simulink library "AEMS_Standard_Library"  (R2016b)
settings: Solver=ode45  StartTime=0.0  StopTime=10.0  RelTol=1e-3
undefined symbols (not defined in the file or in its folder): BkPY, Cbx_extegr, Cbx_lpegrsys, Cbx_portegr, Cnx_bnk_nr_conf, Cnx_cyl_nr_conf, Cxx_dcm_io_tmr_end_xxxx, Cxx_dcm_rt_tmr_end, Cxx_DID_xxxx_IO_max, Cxx_DID_xxxx_IO_min, Cxx_vmaniegi, DEM_DEBOUNCE_FREEZE, DEM_DTR_CTL_INVISIBLE, DEM_DTR_CTL_NORMAL, Dem_DtrId2_XXX, Dem_DtrId3_XXX, Dem_DtrId4_XXX, Dem_DtrId5_XXX, Dem_DtrId6_XXX, Dem_DtrId7_XXX, Dem_DtrId8_XXX, Dem_DtrId9_XXX, Dem_DtrId_XXX, Dem_EnableConditionId2_XXX, Dem_EnableConditionId3_XXX, Dem_EnableConditionId4_XXX, Dem_EnableConditionId5_XXX, Dem_EnableConditionId6_XXX, Dem_EnableConditionId7_XXX, Dem_EnableConditionId8_XXX, Dem_EnableConditionId_XXX, Dem_EventId, Dem_EventId2_XXX, Dem_EventId3_XXX, Dem_EventId4_XXX, Dem_EventId5_XXX, Dem_EventId6_XXX, Dem_EventId7_XXX, Dem_EventId8_XXX, Dem_EventId9_XXX, Dem_EventId_Device_Faulttype, Dem_EventId_XXX, DEM_IUMPR_GENERAL_DENOMINATOR, DEM_OPCYC_IGNITION, Dem_RatioId2_XXX, Dem_RatioId3_XXX, Dem_RatioId4_XXX, Dem_RatioId5_XXX, Dem_RatioId6_XXX, Dem_RatioId7_XXX, Dem_RatioId8_XXX, Dem_RatioId_XXX, Dem_StorageConditionId2_XXX, Dem_StorageConditionId3_XXX, Dem_StorageConditionId4_XXX, Dem_StorageConditionId5_XXX, Dem_StorageConditionId6_XXX, Dem_StorageConditionId7_XXX, Dem_StorageConditionId8_XXX, Dem_StorageConditionId_XXX ... (+14)
undefined symbols (not defined in the file): BreakPoint, Breakpoint, BreakPoint_X, BreakPoint_Y, Cbx_dem_byp_fail_Device_Faulttype, Cbx_dem_jmp_dwn_act_Device_Faulttype, Cbx_dem_jmp_up_act_Device_Faulttype, Cnx_dem_fail_thd_Device_Faulttype, Cnx_dem_jmp_dwn_ppass_Device_Faulttype, Cnx_dem_jmp_up_pfail_Device_Faulttype, Cnx_dem_pass_thd_Device_Faulttype, Cnx_dem_pfail_inc_step_Device_Faulttype, Cnx_dem_ppass_dec_step_Device_Faulttype, Cxb, Cxb_lb_dly_t_para, Cxb_x, Cxb_X, Cxb_y, Cxb_Y, Cxd, Cxm, Cxp, Cxp_lb_a1_1, Cxp_lb_a1_2, Cxp_lb_a1_3, Cxp_lb_a2_1, Cxp_lb_a2_2, Cxp_lb_a2_3, Cxp_lb_b0_1, Cxp_lb_b0_2, Cxp_lb_b0_3, Cxp_lb_b1_1, Cxp_lb_b1_2, Cxp_lb_b1_3, Cxx_dem_fail_thd_Device_Faulttype, Cxx_dem_pass_thd_Device_Faulttype, Cxx_Tol, Cxx_Tol_X, Cxx_Tol_Y, Nnx_dcm_rt_abrt_stt, Nnx_dcm_rt_run_stt, Nxb_fil_para, Nxp_fil_para
libraries: AEMS_Standard_Library x477, simulink x2
(part 1 of 39)
settings Model: ModifiedComment=z021453 -- Mon Apr 01 17:30:33 2019 -- Version $Revision: 2-12 $\nDebugVer:68  Creator=p075121  LastModifiedBy=a002701
settings Model: ModifiedHistory=|
  | AEMS_Standard_Library_02_15_6: by Etienne, Jegan and Caleb, 08-04-2020
  | 
  | 1.AEMS_Standard_Library/DISCONTINUITIES/AEMS_ENUMERATION_SWITCH: Mask Initialisation code updated to avoid block update for inputs, if DataPortIndices is not available in workspace. Icon Drawing Code Updated
  | 
  | AEMS_Standard_Library_02_15_5: by Caleb and Saravana, 01-04-2020
  | 
  | 1.AEMS_Standard_Library/DISCONTINUITIES/AEMS_ENUMERATION_SWITCH: Mask Initialisation code updated to avoid initial loading warning.
  | 
  | AEMS_Standard_Library_02_15_3: by Sindhuja, 20-03-2020
  | 
  | 1.AEMS_Standard_Library/DISCONTINUITIES/AEMS_ENUMERATION_SWITCH: Mask initialisation code is updated to handle multiple constants for single dataport and mask appearance is modified.
  | 2.AEMS_Standard_Library/SPECIFIC/AEMS_SUPPLIER_CALL_ICLC_LEARNING: New supplier call block for ICLC_LEARNING
  | 
  | AEMS_Standard_Library_02_15_2: by Sindhuja, 09-03-2020
  | 
  | 1.AEMS_Standard_Library/DISCONTINUITIES/AEMS_ENUMERATION_SWITCH: Custom multiport switch block to display enum constant names on the mask.
  | 2.AEMS_Standard_Library/DCM/AEMS_DCM_DID_WRITEDATA:Deletion of NVM WriteOnFly settings.
  | 
  | AEMS_Standard_Library_02_15_1: by Sindhuja, 04-03-2020
  | 
  | 1.Naming convention of Bus Signal wire names are reverted to Uppercase "Index" and "Ratio" [AUTOSAR Constraint] for the below blocks.
  | AEMS_Standard_Library/LOOKUP_TABLES/AEMS_DIRECTLU_1D
  | AEMS_Standard_Library/LOOKUP_TABLES/AEMS_DIRECTLU_2D
  | AEMS_Standard_Library/LOOKUP_TABLES/AEMS_DIRECTLU_INDEXED_1D
  | AEMS_Standard_Library/LOOKUP_TABLES/AEMS_DIRECTLU_INDEXED_2D
  | 
  | 2.To display EventId as eventid in the Attribute format string as per the MXAM guidelines. And added new raster suffix to “DataStoreName” and now the code is generalised to add any type of new raster suffix in the below blocks.
  | AEMS_Standard_Library/DEM/AEMS_DEM_COUNTER_BASED_DEBOUNCE_THRSHOLD_DYN
  | AEMS_Standard_Library/DEM/AEMS_DEM_TIME_BASED_DEBOUNCE_THRSHOLD_DYN
  | 
  | 3.Added new raster suffix to “DataStoreName” and now the code is generalised to add any type of new raster suffix.
  | "AEMS_Standard_Library/SPECIFIC/" : 89 Supplier call blocks
  | AEMS_Standard_Library/SUB/AEMS_DEM_GETEVENTSTATUS
  | AEMS_Standard_Library/SUB/AEMS_FIM_GETFUNCTIONPERMISSION
  | AEMS_Standard_Library/DEM/AEMS_DEM_COUNTER_BASED_DEBOUNCE
  | AEMS_Standard_Library/DEM/AEMS_DEM_TIME_BASED_DEBOUNCE
  | AEMS_Standard_Library_02_15_0: by Sindhuja, 14-02-2020
  | 
  | 1.AEMS_Standard_Library/LOOKUP_TABLES/AEMS_PRE_INTERP: Naming convention of Bus Signal wire names are reverted to Uppercase "Index" and "Ratio" [AUTOSAR Constraint]
  | 
  | To avoid underspecified datatype warnings, stronger typing of the datatypes are done in the below library blocks:
  | 1.AEMS_Standard_Library/DCM/AEMS_APP_REQUEST_ROUTINE:The Output Datatype of the following blocks is strongly typed as "single" in "AEMS_APP_REQUEST_ROUTINE/Timer_routine_Subsystem/" Product,Divide,Sum blocks.
  | 2.AEMS_Standard_Library/DCM/AEMS_DCM_REQUEST_RESULT/Callback_Subsystem/Add:Output Datatype is strongly typed as “uint8”.
  | 3.AEMS_Standard_Library/DCM/AEMS_APP_REQUEST_IOCONTROL/Timer_IOControl_Subsystem/Sum:Output Datatype of the sum block is strongly typed as "single".
  | 4.AEMS_Standard_Library/DCM/AEMS_DCM_START_ROUTINE/Callback_Subsystem/Add:Output Datatype for the above block should be strongly typed as “uint8”.
  | 5.AEMS_Standard_Library/DCM/AEMS_DCM_STOP_ROUTINE/Xxx_Stop_Callback/Add:Output Datatype for the above block is strongly typed as “uint8”.
  | 6.AEMS_Standard_Library/TIMER/AEMS_TIMER1:Output Datatype of the constant blocks are strongly typed as "single" for Constant1,Constant2,Constant3,Constant4,Constant5 blocks.
  | 
  | AEMS_Standard_Library_02_14_2: by Sindhuja, 28-11-2019
  | 
  | 1.AEMS_Standard_Library/LOOKUP_TABLES/AEMS_ITP3D: Block is migrated from RSA_Itp3D for computing 3D interpolation
  | 2.AEMS_Standard_Library/DEM/AEMS_DEM_REP_IUMPR: The background colour of the block is made red as the block is obsolete
  | 3.AEMS_Standard_Library/DCM/AEMS_DCM_DID_WRITEDATA: Optimization of the Mask Initialization code
  | 4.AEMS_Standard_Library/DCM/AEMS_DCM_IO_SHORT_TERM_ADJUSTMENT: Optimization of the Mask Initialization code
  | 5.AEMS_Standard_Library/DEM/AEMS_DEM_SET_EVENT_STS: Default dimension of the block is set as "1“ when the Specific case for Nissan is “on”
  | 6.AEMS_Standard_Library/DEM/AEMS_DEM_SET_DTR: Default dimension of the block is set as "1“ when the Specific case for Nissan is “on”
  | 
  | AEMS_Standard_Library_02_13_13: by Sindhuja, 18-10-2019
  | 
  | 1. AEMS_Standard_Library/DCM/AEMS_DCM_IO_SHORT_TERM_ADJUSTMENT: DataType “Boolean” is added in parameter DID_DataType.
  |   The output datatype of the constant blocks “Cxx_DID_xxxx_IO_max” and “Cxx_DID_xxxx_IO_min” is set to “Inherit via back propagation”.
  | 2. AEMS_Standard_Library/MATH/AEMS_PROTECTED_DIVISION: Block has been updated to take care of vector denominator.
  | 3. Graphical changes(Default size) of these blocks are made as same as that of REMS:
  |    AEMS_Standard_Library/FLAG/AEMS_SRFLIPFLOP
  |    AEMS_Standard_Library/EDGE/AEMS_EDGE_EITHER
  |    AEMS_Standard_Library/EDGE/AEMS_EDGE_FALLING
  |    AEMS_Standard_Library/EDGE/AEMS_EDGE_RISING
  | 
  | AEMS_Standard_Library_02_13_12 : by Smriti, 09-10-2019
  | 
  | 1. AEMS_Standard_Library/DCM/ AEMS_DCM_DID_WRITEDATA: Adding Datatype convert block between “Conversion_Subsystem” blocks and “DID_” blocks.
  | 2. In Data Store Write block, “DataStoreName” is updated according to the “EventId” followed by the raster suffix.
  | AEMS_Standard_Library/DEM/AEMS_DEM_COUNTER_BASED_DEBOUNCE
  | AEMS_Standard_Library/DEM/AEMS_DEM_COUNTER_BASED_DEBOUNCE_THRSHOLD_DYN
  | AEMS_Standard_Library/DEM/AEMS_DEM_TIME_BASED_DEBOUNCE
  | AEMS_Standard_Library/DEM/AEMS_DEM_TIME_BASED_DEBOUNCE_THRSHOLD_DYN
  | 
  | 3. The data type for the constant blocks present in the below listed AEMS blocks is set as "inherit from constant value" for the following blocks:
  | DemDebounceCounterFailedThreshold
  | DemDebounceCounterIncrementStepSize
  | DemDebounceCounterJumpUp
  | DemDebounceCounterJumpUpValue
  | DebounceCounterPassedThreshold
  | DemDebounceCounterDecrementStepSize
  | DemDebounceCounterJumpDown
  | DemDebounceCounterJumpDownValue
  | 
  | AEMS  Library blocks:
  | AEMS_Standard_Library/SUB/AEMS_DEM_COUNTER_BASED_DEBOUNCE_1D
  | AEMS_Standard_Library/SUB/AEMS_DEM_COUNTER_BASED_DEBOUNCE_2D
  | AEMS_Standard_Library/SUB/AEMS_DEM_COUNTER_BASED_DEBOUNCE_3D
  | AEMS_Standard_Library/SUB/AEMS_DEM_COUNTER_BASED_DEBOUNCE_4D
  | AEMS_Standard_Library/SUB/AEMS_DEM_COUNTER_BASED_DEBOUNCE_6D
  | AEMS_Standard_Library/SUB/AEMS_DEM_COUNTER_BASED_DEBOUNCE_8D
  | AEMS_Standard_Library/SUB/AEMS_DEM_COUNTER_BASED_DEBOUNCE_THRSHOLD_DYN_1D
  | AEMS_Standard_Library/SUB/AEMS_DEM_COUNTER_BASED_DEBOUNCE_THRSHOLD_DYN_2D
  | AEMS_Standard_Library/SUB/AEMS_DEM_COUNTER_BASED_DEBOUNCE_THRSHOLD_DYN_3D
  | AEMS_Standard_Library/SUB/AEMS_DEM_COUNTER_BASED_DEBOUNCE_THRSHOLD_DYN_4D
  | AEMS_Standard_Library/SUB/AEMS_DEM_COUNTER_BASED_DEBOUNCE_THRSHOLD_DYN_6D
  | AEMS_Standard_Library/SUB/AEMS_DEM_COUNTER_BASED_DEBOUNCE_THRSHOLD_DYN_8D
  | AEMS_Standard_Library/SUB/AEMS_DEM_TIME_BASED_DEBOUNCE_1D
  | AEMS_Standard_Library/SUB/AEMS_DEM_TIME_BASED_DEBOUNCE_2D
  | AEMS_Standard_Library/SUB/AEMS_DEM_TIME_BASED_DEBOUNCE_3D
  | AEMS_Standard_Library/SUB/AEMS_DEM_TIME_BASED_DEBOUNCE_4D
  | AEMS_Standard_Library/SUB/AEMS_DEM_TIME_BASED_DEBOUNCE_6D
  | 
  | AEMS_Standard_Library_02_13_11 : by Sindhuja, 30-09-2019
  | 
  | 1. AEMS_Standard_Library/MATH/AEMS_COUNTER: The logical implementation has been modified so as to take care when the transition of start_flag from 1 to 0 after saturation occurs at 255.
  | 2. AEMS_Standard_Library/COM/AEMS_FRAME_SUPERVISION:The AEMS_NVM_SET block has been replaced by the unit delay block and vice versa.The Status of the block is sent to unit delay instead of AEMS_NVM_SET in “AEMS_FRAME_SUPERVISION”.
  |     And the Frame_Detected previous value is now sent to AEMS_NVM_SET instead of the unit delay in “AEMS_FRAME_SUPERVISION/ecu_frm_detection”.
  | 3. AEMS_Standard_Library/MEM/AEMS_NVM_WRITEONFLY:Parameter for TriggerType (Rising Edge or Enable) is added.
  |    The  block “AEMS_NVM_WRITEONFLY_ENABLE” is made obsolete.
  | 4. AEMS_Standard_Library/SUB/AEMS_DEM_REPIUMPRDENRELEASE: The attribute format string "sample time" for the "ratioid" is removed.
  |     Dem_RepIUMPRDenLock with the rising edge is removed and the Dem_RepIUMPRDenRelease with the falling edge is replaced with the rising edge in all these blocks.
  |     AEMS_DEM_REP_IUMPR_DEN_RELEASE_1D
  |     AEMS_DEM_REP_IUMPR_DEN_RELEASE_2D
  |     AEMS_DEM_REP_IUMPR_DEN_RELEASE_8D
  | 5. AEMS_Standard_Library/DCM/AEMS_DCM_DID_WRITEDATA: Updated the Initialisation code to set the “TriggerType” of the child library “AEMS_NVM_WRITEONFLY” to “Enable”.
  | 6. AEMS_Standard_Library/DEM/AEMS_FIM_GETFUNCTIONINHIBITION: The constant block “FID_Block” in the below child blocks is set to datatype “uint8”.
  |     AEMS_Standard_Library/SUB/AEMS_FIM_GETFUNCTIONPERMISSION
  |     AEMS_Standard_Library/SUB/AEMS_FIM_GET_FUNC_PMT_1D
  |     AEMS_Standard_Library/SUB/AEMS_FIM_GET_FUNC_PMT_2D
  | 7. AEMS_Standard_Library/SUB/AEMS_FIM_GET_FUNC_PMT_2D: The FIM fid naming has been changed as Fim_fid_xxxx_1 and Fim_fid_xxxx_2
  | 
  | AEMS_Standard_Library_02_13 : by Sindhuja, 18-09-2019
  | 
  | The following blocks are updated with below requirements,
  | -	C**_<Default>_<Faultype> parameters gets updated based on the changes in EventId.
  | -	Additional input “ClearDataRequest” is added.
  | -	New parameter “Cbx_dem_byp_fail_device_faulttype” is added.
  | -	Write output To DataStoreMemory mode added.
  | 
  | 1. AEMS_Standard_Library/DEM/AEMS_DEM_TIME_BASED_DEBOUNCE
  | 2. AEMS_Standard_Library/DEM/AEMS_DEM_COUNTER_BASED_DEBOUNCE
  | 3. AEMS_Standard_Library/DEM/AEMS_DEM_COUNTER_BASED_DEBOUNCE_THRSHOLD_DYN
  | 4. AEMS_Standard_Library/DEM/AEMS_DEM_TIME_BASED_DEBOUNCE_THRSHOLD_DYN
  | 5. AEMS_Standard_Library/SUB/AEMS_DEM_COUNTERBASEDDEBOUNCE
  | 6. AEMS_Standard_Library/SUB/AEMS_DEM_COUNTER_BASED_DEBOUNCE_1D
  | 7. AEMS_Standard_Library/SUB/AEMS_DEM_COUNTER_BASED_DEBOUNCE_2D
  | 8. AEMS_Standard_Library/SUB/AEMS_DEM_COUNTER_BASED_DEBOUNCE_3D
  | 9. AEMS_Standard_Library/SUB/AEMS_DEM_COUNTER_BASED_DEBOUNCE_4D
  | 10. AEMS_Standard_Library/SUB/AEMS_DEM_COUNTER_BASED_DEBOUNCE_6D
  | 11. AEMS_Standard_Library/SUB/AEMS_DEM_COUNTER_BASED_DEBOUNCE_8D
  | 12.AEMS_Standard_Library/SUB/AEMS_DEM_COUNTER_BASED_DEBOUNCE_THRSHOLD_DYN_1D
  | 13.AEMS_Standard_Library/SUB/AEMS_DEM_COUNTER_BASED_DEBOUNCE_THRSHOLD_DYN_2D
  | 14.AEMS_Standard_Library/SUB/AEMS_DEM_COUNTER_BASED_DEBOUNCE_THRSHOLD_DYN_3D
  | 15.AEMS_Standard_Library/SUB/AEMS_DEM_COUNTER_BASED_DEBOUNCE_THRSHOLD_DYN_4D
  | 16.AEMS_Standard_Library/SUB/AEMS_DEM_COUNTER_BASED_DEBOUNCE_THRSHOLD_DYN_6D
  | 17.AEMS_Standard_Library/SUB/AEMS_DEM_COUNTER_BASED_DEBOUNCE_THRSHOLD_DYN_8D
  | 18.AEMS_Standard_Library/SUB/AEMS_DEM_TIMEBASEDDEBOUNCE
  | 19.AEMS_Standard_Library/SUB/AEMS_DEM_TIME_BASED_DEBOUNCE_1D
  | 20.AEMS_Standard_Library/SUB/AEMS_DEM_TIME_BASED_DEBOUNCE_2D
  | 21.AEMS_Standard_Library/SUB/AEMS_DEM_TIME_BASED_DEBOUNCE_3D
  | 22.AEMS_Standard_Library/SUB/AEMS_DEM_TIME_BASED_DEBOUNCE_4D
  | 23.AEMS_Standard_Library/SUB/AEMS_DEM_TIME_BASED_DEBOUNCE_6D
  | 24.AEMS_Standard_Library/SUB/AEMS_DEM_TIME_BASED_DEBOUNCE_8D
  | 25.AEMS_Standard_Library/SUB/AEMS_DEM_TIME_BASED_DEBOUNCE_THRSHOLD_DYN_1D
  | 26.AEMS_Standard_Library/SUB/AEMS_DEM_TIME_BASED_DEBOUNCE_THRSHOLD_DYN_2D
  | 27.AEMS_Standard_Library/SUB/AEMS_DEM_TIME_BASED_DEBOUNCE_THRSHOLD_DYN_3D
  | 28.AEMS_Standard_Library/SUB/AEMS_DEM_TIME_BASED_DEBOUNCE_THRSHOLD_DYN_4D
  | 29.AEMS_Standard_Library/SUB/AEMS_DEM_TIME_BASED_DEBOUNCE_THRSHOLD_DYN_6D
  | 30.AEMS_Standard_Library/SUB/AEMS_DEM_TIME_BASED_DEBOUNCE_THRSHOLD_DYN_8D
  | 
  | 31.AEMS_Standard_Library/DCM/AEMS_DCM_DID_WRITEDATA:
  | -	Parameter name has been changed from “DID Datatype” to “DID Monitoring Datatype”.
  | -	When NVM WriteOnFly Variables is ON, the output of each DID will be tapped into an input of the AEMS_NVM_WRITEONFLY block.
  | -	According to the New rule ARS_STP, the sample time of the constant blocks are set as "inf" in these blocks: AEMS_DCM_DID_WRITEDATA/Callback_Subsystem/..Constant3,
  | 	Constant2, Constant1, NRC1.
  | 
  | 32.AEMS_Standard_Library/MEM/AEMS_NVM_WRITEONFLY: Block is updated to throw an error when the “Number of Inputs” is zero.
  | 33.AEMS_Standard_Library/MATH/AEMS_PROTECTED_DIVISION: New block that replaces the block AEMS_DIVISION_BY_ZERO with a new parameter "Output when |Denominator| < Tolerance".
  |    AEMS_DIVISION_BY_ZERO block is made obsolete. So use AEMS_PROTECTED_DIVISION instead.
  | 34.AEMS_Standard_Library/SUB/AEMS_DEADZONE: The functional implementation has been modified to match REMS behaviour.Block is moved from category "SUB" to "DISCONTINUITIES"
  | 35.AEMS_Standard_Library/DEM/AEMS_DEM_GET_INDICATOR_STS: New parameter for "Simulation Mode" is added.
  | 36.AEMS_Standard_Library/SUB/AEMS_DEM_GETINDICATORSTATUS: New parameter for "Simulation Mode" is added.
  | 37.AEMS_Standard_Library/MATH/AEMS_MATRIX_INVERSION: New block to compute the inversion of a 3*3 matrix.
  | 38.AEMS_Standard_Library/LOOKUP_TABLES/AEMS_INDEXED_LUT_1D_TOL: Newly added block equivalent to RSA_Index_1D_Tol_v01_02
  | 
  | Updated the raster suffix to be added for “DataStoreName” in the “DataStoreRead” block and the constant block “FID block” is set to datatype “uint32” in the below blocks.
  | 39.AEMS_Standard_Library/SUB/AEMS_FIM_GETFUNCTIONPERMISSION
  | 40.AEMS_Standard_Library/SUB/AEMS_FIM_GET_FUNC_PMT_1D
  | 41.AEMS_Standard_Library/SUB/AEMS_FIM_GET_FUNC_PMT_2D
  | 42.AEMS_Standard_Library/DEM/AEMS_FIM_GETFUNCTIONINHIBITION
  | 
  | 43."AEMS_Standard_Library/SPECIFIC/" : 89 Supplier call blocks are updated  under this category: The raster suffix gets added for the “DataStoreName” in the “DataStoreRead” block with respect to the function call trigger.
  | 44.AEMS_Standard_Library/SAFETY/AEMS_SAFETY_AND_REGULATION: To insure traceability of Safety and Regulation requirements, new block AEMS_SAFETY_AND_REGULATION is added.
  | 
  | The parameter case has been changed from Dem_StorageConditionID to "Dem_StorageConditionId" in the below blocks.
  | 45.AEMS_Standard_Library/DEM/AEMS_DEM_SET_STORAGE_COND
  | 46.AEMS_Standard_Library/SUB/AEMS_DEM_SET_STORAGE_COND_2D
  | 47.AEMS_Standard_Library/DEM/AEMS_DEM_SET_STORAGE_COND_3D
  | 48.AEMS_Standard_Library/DEM/AEMS_DEM_SET_STORAGE_COND_8D
  | 
  | 49.AEMS_Standard_Library/DCM/AEMS_DCM_IO_SHORT_TERM_ADJUSTMENT: Block spelling is corrected from AEMS_DCM_IO_SHORT_TERM_ADJUSTEMENT to AEMS_DCM_IO_SHORT_TERM_ADJUSTMENT
  | 50.AEMS_Standard_Library/SUB/AEMS_SORT_MEDIAN: "AEMS_SORT_MEDIAN/Pair/Add1" here "Require all inputs to have same datatype" and "Saturate on integer overflow" has been enabled.
  | 51.AEMS_Standard_Library/DISCRETE/AEMS_UNITDELAY_RESET_EXTERNALIC: The wire names has been removed for inports 2 and 3.
  | 52.AEMS_Standard_Library/FILTER/AEMS_FIRST_ORDER_FILTER_RST: Stronger typing of DataTypes of Sum, Sum1, Product1 and Product2 blocks are changed to “single” to avoid warnings.
  | 
  | 
  | AEMS_Standard_Library_02_12 : by Sindhuja, 21-06-2019
  | 
  | New parameter "Function Mode" is added for DSM possibility in the following blocks:
  | 1. AEMS_Standard_Library/DEM/AEMS_DEM_GET_EVENT_STS
  | 2. AEMS_Standard_Library/SUB/AEMS_DEM_GETEVENTSTATUS
  | 3. AEMS_Standard_Library/SUB/AEMS_DEM_GET_EVENT_STS_1D
  | 4. AEMS_Standard_Library/SUB/AEMS_DEM_GET_EVENT_STS_2D
  | 5. AEMS_Standard_Library/SUB/AEMS_DEM_GET_EVENT_STS_8D
  | 6. AEMS_Standard_Library/SUB/AEMS_DEM_GET_EVENT_STS_9D
  | 
  | 7. AEMS_Standard_Library/BIT_OPERATION/AEMS_BIT_SET32: New Library block
  | 
  | 8. AEMS_Standard_Library/MATH/AEMS_SORT: New Library block to sort one-dimensional arrays
  | 9. AEMS_Standard_Library/SUB /AEMS_SORT_MEDIAN: Child library for AEMS_SORT, to get the median vector after sorting the N numbers in ascending order.
  | 
  | 10. AEMS_Standard_Library/MATH/AEMS_SORT:Implementation has been modified in "AEMS_SORT/For_loop_1/For_loop_2/Unit_delay_vector"
  | 
  | AEMS_Standard_Library_02_12 : by Sindhuja, 06-06-2019
  | "Dem debounce behavior 1" is set to "DEM_DEBOUNCE_FREEZE" by default for the following blocks:
  | 1. AEMS_Standard_Library/DEM/AEMS_DEM_TIME_BASED_DEBOUNCE
  | 2. AEMS_Standard_Library/DEM/AEMS_DEM_COUNTER_BASED_DEBOUNCE
  | 3. AEMS_Standard_Library/DEM/AEMS_DEM_TIME_BASED_DEBOUNCE_THRSHOLD_DYN
  | 
  | 4. AEMS_Standard_Library/SUB/AEMS_DEM_SET_STORAGE_COND_1D: The Output Datatype of StorageCondId is set to uint8
  | 5. AEMS_Standard_Library/SUB/AEMS_DEM_REP_IUMPR_1D: The Output Datatype of RatioId is set to uint16
  | 6. AEMS_Standard_Library/SUB/AEMS_DEM_REP_IUMPR_2D: The Output Datatype of RatioId is set to uint16
  | 7. AEMS_Standard_Library/SUB/AEMS_DEM_REP_IUMPR_DEN_RELEASE_1D: The Output Datatype of RatioId is set to uint16
  | 8. AEMS_Standard_Library/SUB/AEMS_DEM_REP_IUMPR_DEN_RELEASE_2D: The Output Datatype of RatioId is set to uint16
  | 9. AEMS_Standard_Library/SUB/AEMS_DEM_REP_IUMPR_FAULTDETECT_1D: The Output Datatype of RatioId is set to uint16
  | 10. AEMS_Standard_Library/SUB/AEMS_DEM_REP_IUMPR_FAULTDETECT_2D: The Output Datatype of RatioId is set to uint16
  | 11. AEMS_Standard_Library/SUB/AEMS_DEM_SET_EVENT_DSBL_1D: The Output Datatype of EventId is set to uint16
  | 12. AEMS_Standard_Library/SUB/AEMS_DEM_GET_EVENT_STS_1D: The Output Datatype of EventId is set to uint16
  | 
  | 
  | AEMS_Standard_Library_02_12 : by Sindhuja, 24-05-2019
  | 1.AEMS_Standard_Library/MATH/AEMS_SQRT: Added option for reciprocal square root in the "Function of Sqrt"
  | 2.AEMS_Standard_Library/DEM/AEMS_FIM_GETFUNCTIONINHIBITION: Updated AEMS_FIM_GetFunctionInhibition to add DSM possibility
  | 3.AEMS_Standard_Library/SUB/AEMS_FIM_GETFUNCTIONPERMISSION: Added DSM possibility
  | 4.AEMS_Standard_Library/SUB/AEMS_FIM_GET_FUNC_PMT_1D: Added DSM possibility
  | 5.AEMS_Standard_Library/SUB/AEMS_FIM_GET_FUNC_PMT_2D: Added DSM possibility
  | 6.New blocks migrated from NEMS to "AEMS_Standard_Library/SPECIFIC"
  |  AEMS_AIR_BALANCE
  |  AEMS_BACK_UP
  |  AEMS_BACK_UP_AVE
  |  AEMS_BACKUP_FOR_ENGINE_OFF_MONITOR
  |  AEMS_DGNDMDPGCUT
  |  AEMS_DGN_MF_MISX_CALCULATION_LIB
  |  AEMS_UL_INTERP
  |  AEMS_INTERP_WITH_BREAKPOINT
  |  AEMS_LOOKUP_LIBRARY
  |  AEMS_EGR_OFFSET_BLOCK_DIM8
  |  AEMS_EGR_RATE_TRANSPORTOR_LIB
  |  AEMS_OL_RATE_COUNTER
  |  AEMS_OL_SIMILAR_CONDITION_SET
  |  AEMS_STATE_TRANSITION_SET_VALUE
  |  AEMS_OL_RATE_COUNTER_B
  |  AEMS_OL_SIMILAR_CONDITION_CHECK
  |  AEMS_EGR_RESPONSE_TIME_CAL_LIB
  |  AEMS_EGRQESTH_SELECT_AND_TRIM_LIB
  |  AEMS_DGN_BB_RESULT
  | 
  |  7.EventId Numbering changed for the below blocks:
  |  AEMS_Standard_Library/SUB/AEMS_DEM_COUNTER_BASED_DEBOUNCE_THRSHOLD_DYN_2D
  |  AEMS_Standard_Library/SUB/AEMS_DEM_COUNTER_BASED_DEBOUNCE_THRSHOLD_DYN_3D
  |  AEMS_Standard_Library/SUB/AEMS_DEM_COUNTER_BASED_DEBOUNCE_THRSHOLD_DYN_4D
  |  AEMS_Standard_Library/SUB/AEMS_DEM_COUNTER_BASED_DEBOUNCE_THRSHOLD_DYN_6D
  |  AEMS_Standard_Library/SUB/AEMS_DEM_COUNTER_BASED_DEBOUNCE_THRSHOLD_DYN_8D
  |  AEMS_Standard_Library/SUB/AEMS_DEM_TIME_BASED_DEBOUNCE_THRSHOLD_DYN_2D
  |  AEMS_Standard_Library/SUB/AEMS_DEM_TIME_BASED_DEBOUNCE_THRSHOLD_DYN_3D
  |  AEMS_Standard_Library/SUB/AEMS_DEM_TIME_BASED_DEBOUNCE_THRSHOLD_DYN_4D
  |  AEMS_Standard_Library/SUB/AEMS_DEM_TIME_BASED_DEBOUNCE_THRSHOLD_DYN_6D
  |  AEMS_Standard_Library/SUB/AEMS_DEM_TIME_BASED_DEBOUNCE_THRSHOLD_DYN_8D
  |  AEMS_Standard_Library/SUB/AEMS_DEM_TIME_BASED_DEBOUNCE_2D
  |  AEMS_Standard_Library/SUB/AEMS_DEM_TIME_BASED_DEBOUNCE_3D
  |  AEMS_Standard_Library/SUB/AEMS_DEM_TIME_BASED_DEBOUNCE_4D
  |  AEMS_Standard_Library/SUB/AEMS_DEM_TIME_BASED_DEBOUNCE_6D
  |  AEMS_Standard_Library/SUB/AEMS_DEM_TIME_BASED_DEBOUNCE_8D
  |  AEMS_Standard_Library/SUB/AEMS_DEM_COUNTER_BASED_DEBOUNCE_2D
  |  AEMS_Standard_Library/SUB/AEMS_DEM_COUNTER_BASED_DEBOUNCE_3D
  |  AEMS_Standard_Library/SUB/AEMS_DEM_COUNTER_BASED_DEBOUNCE_4D
  |  AEMS_Standard_Library/SUB/AEMS_DEM_COUNTER_BASED_DEBOUNCE_6D
  |  AEMS_Standard_Library/SUB/AEMS_DEM_COUNTER_BASED_DEBOUNCE_8D
  |  AEMS_Standard_Library/SUB/AEMS_DEM_SET_STORAGE_COND_2D
  |  AEMS_Standard_Library/SUB/AEMS_DEM_SET_STORAGE_COND_8D
  |  AEMS_Standard_Library/SUB/AEMS_DEM_REP_IUMPR_2D
  |  AEMS_Standard_Library/SUB/AEMS_DEM_REP_IUMPR_8D
  |  AEMS_Standard_Library/SUB/AEMS_DEM_REP_IUMPR_DEN_RELEASE_2D
  |  AEMS_Standard_Library/SUB/AEMS_DEM_REP_IUMPR_DEN_RELEASE_8D
  |  AEMS_Standard_Library/SUB/AEMS_DEM_REP_IUMPR_FAULTDETECT_2D
  |  AEMS_Standard_Library/SUB/AEMS_DEM_REP_IUMPR_FAULTDETECT_8D
  |  AEMS_Standard_Library/SUB/AEMS_DEM_SET_EVENT_DSBL_2D
  |  AEMS_Standard_Library/SUB/AEMS_DEM_SET_EVENT_DSBL_8D
  |  AEMS_Standard_Library/SUB/AEMS_DEM_SET_EVENT_DSBL_9D
  |  AEMS_Standard_Library/SUB/AEMS_DEM_GET_EVENT_STS_2D
  |  AEMS_Standard_Library/SUB/AEMS_DEM_GET_EVENT_STS_8D
  |  AEMS_Standard_Library/SUB/AEMS_DEM_GET_EVENT_STS_9D
  |  AEMS_Standard_Library/SUB/AEMS_DEM_SET_EVENT_STS_2D
  |  AEMS_Standard_Library/SUB/AEMS_DEM_SET_EVENT_STS_8D
  |  AEMS_Standard_Library/SUB/AEMS_DEM_SET_EVENT_STS_9D
  |  AEMS_Standard_Library/SUB/AEMS_DEM_SET_EVENT_AVL_2D
  |  AEMS_Standard_Library/SUB/AEMS_DEM_SET_EVENT_AVL_8D
  |  AEMS_Standard_Library/SUB/AEMS_DEM_SET_EVENT_AVL_9D
  |  AEMS_Standard_Library/SUB/AEMS_FIM_GET_FUNC_PMT_2D
  |  AEMS_Standard_Library/SUB/AEMS_DEM_SET_ENBL_COND_2D
  |  AEMS_Standard_Library/SUB/AEMS_DEM_SET_ENBL_COND_8D
  |  AEMS_Standard_Library/SUB/AEMS_DEM_SET_DTR_2DS
  |  AEMS_Standard_Library/SUB/AEMS_DEM_SET_DTR_8DS
  |  AEMS_Standard_Library/SUB/AEMS_DEM_SET_DTR_2DU
  |  AEMS_Standard_Library/SUB/AEMS_DEM_SET_DTR_8DU
  |  AEMS_Standard_Library/SUB/AEMS_DEM_SET_DTR_9DU
  | 
  |  8.Changed EventID to EventId in the below blocks:
  |  AEMS_Standard_Library/DEM/AEMS_DEM_SET_EVENT_AVL
  |  AEMS_Standard_Library/DEM/AEMS_DEM_TIME_BASED_DEBOUNCE
  |  AEMS_Standard_Library/DEM/AEMS_DEM_COUNTER_BASED_DEBOUNCE
  |  AEMS_Standard_Library/DEM/AEMS_DEM_TIME_BASED_DEBOUNCE_THRSHOLD_DYN
  |  AEMS_Standard_Library/DEM/AEMS_DEM_COUNTER_BASED_DEBOUNCE_THRSHOLD_DYN
  |  AEMS_Standard_Library/SUB/AEMS_DEM_TIMEBASEDDEBOUNCE
  |  AEMS_Standard_Library/SUB/AEMS_DEM_COUNTERBASEDDEBOUNCE
  |  AEMS_Standard_Library/SUB/AEMS_DEM_COUNTER_BASED_DEBOUNCE_THRSHOLD_DYN_1D
  |  AEMS_Standard_Library/SUB/AEMS_DEM_COUNTER_BASED_DEBOUNCE_THRSHOLD_DYN_2D
  |  AEMS_Standard_Library/SUB/AEMS_DEM_COUNTER_BASED_DEBOUNCE_THRSHOLD_DYN_3D
  |  AEMS_Standard_Library/SUB/AEMS_DEM_COUNTER_BASED_DEBOUNCE_THRSHOLD_DYN_4D
  |  AEMS_Standard_Library/SUB/AEMS_DEM_COUNTER_BASED_DEBOUNCE_THRSHOLD_DYN_6D
  |  AEMS_Standard_Library/SUB/AEMS_DEM_COUNTER_BASED_DEBOUNCE_THRSHOLD_DYN_8D
  |  AEMS_Standard_Library/SUB/AEMS_DEM_TIME_BASED_DEBOUNCE_THRSHOLD_DYN_1D
  |  AEMS_Standard_Library/SUB/AEMS_DEM_TIME_BASED_DEBOUNCE_THRSHOLD_DYN_2D
  |  AEMS_Standard_Library/SUB/AEMS_DEM_TIME_BASED_DEBOUNCE_THRSHOLD_DYN_3D
  |  AEMS_Standard_Library/SUB/AEMS_DEM_TIME_BASED_DEBOUNCE_THRSHOLD_DYN_4D
  |  AEMS_Standard_Library/SUB/AEMS_DEM_TIME_BASED_DEBOUNCE_THRSHOLD_DYN_6D
  |  AEMS_Standard_Library/SUB/AEMS_DEM_TIME_BASED_DEBOUNCE_THRSHOLD_DYN_8D
  |  AEMS_Standard_Library/SUB/AEMS_DEM_TIME_BASED_DEBOUNCE_1D
  |  AEMS_Standard_Library/SUB/AEMS_DEM_TIME_BASED_DEBOUNCE_2D
  |  AEMS_Standard_Library/SUB/AEMS_DEM_TIME_BASED_DEBOUNCE_3D
  |  AEMS_Standard_Library/SUB/AEMS_DEM_TIME_BASED_DEBOUNCE_4D
  |  AEMS_Standard_Library/SUB/AEMS_DEM_TIME_BASED_DEBOUNCE_6D
  |  AEMS_Standard_Library/SUB/AEMS_DEM_TIME_BASED_DEBOUNCE_8D
  |  AEMS_Standard_Library/SUB/AEMS_DEM_COUNTER_BASED_DEBOUNCE_1D
  |  AEMS_Standard_Library/SUB/AEMS_DEM_COUNTER_BASED_DEBOUNCE_2D
  |  AEMS_Standard_Library/SUB/AEMS_DEM_COUNTER_BASED_DEBOUNCE_3D
  |  AEMS_Standard_Library/SUB/AEMS_DEM_COUNTER_BASED_DEBOUNCE_4D
  |  AEMS_Standard_Library/SUB/AEMS_DEM_COUNTER_BASED_DEBOUNCE_6D
  |  AEMS_Standard_Library/SUB/AEMS_DEM_COUNTER_BASED_DEBOUNCE_8D
  | 
  | 9.AEMS_Standard_Library/LOOKUP_TABLES/AEMS_PRE_INTERP:Naming of the wires is made to lower case
  | 10.AEMS_Standard_Library/SUB/AEMS_DEM_READDATAOFPID01:Signal name “vPID01” is removed inside the library block
  | 11.AEMS_Standard_Library/SUB/AEMS_DEM_SET_DTR_1DU: The Output Datatype for the constant blocks DEM_DTR_CTL_NORMAL & DEM_DTR_CTL_INVISIBLE is changed from "inherit from constant value" to “uint8”
  | 12.AEMS_Standard_Library/SUB/AEMS_DEM_SET_DTR_2DU: The Output Datatype for the constant blocks DEM_DTR_CTL_NORMAL & DEM_DTR_CTL_INVISIBLE is changed from "inherit from constant value" to “uint8”
  | 13.AEMS_Standard_Library/TIMER/AEMS_TIMER: No functional changes. Stronger typing of Datatypes to avoid Underspecified warnings.
  | 14.AEMS_Standard_Library/DCM/AEMS_DCM_IO_SHORT_TERM_ADJUSTEMENT:  The parameter DataSize is replaced by DataType(int8/uint8/int16/uint16/int32/uint32).
  |      Changes done in the “Mask initialization” for the replace block command. A demux block is added to handle if buffer size is 2byte or 4byte.
  | 15.AEMS_Standard_Library/DCM/AEMS_DCM_DID_WRITEDATA:Input is removed and Ground is added.
  | 16.AEMS_Standard_Library/SAFETY/AEMS_FSL_RAM_QM_TO_ASIL: Nissan Safety block
  | 17.AEMS_Standard_Library/SAFETY/AEMS_FSL_RAM_ASIL_TO_QM: Nissan Safety block
  | 18.AEMS_Standard_Library/FILTER/AEMS_TAU_TO_FILTER_PARAM_EXP: An obsolete block for Prefilter with exponential.
  | 
  | AEMS_Standard_Library_02_11 : by Sindhuja, 18-03-2019
  | 1. AEMS_Standard_Library/SUB/AEMS_CONVERT_BUFFER_TO_FLP: Data Type Conversion block added in the library block "AEMS_CONVERT_BUFFER_TO_FLP".
  | 2. AEMS_Standard_Library/DCM/AEMS_DCM_DID_WRITEDATA: Updated the child library block "AEMS_CONVERT_BUFFER_TO_FLP" in "AEMS_DCM_DID_WRITEDATA".
  | 3. AEMS_Standard_Library/DCM/AEMS_FLOAT_TO_FXP: Internal implementation doesn’t have Min/Max Limits. And the parameter "ByteSize" has been changed to "Output Fixed Point datatype".
  | 4. AEMS_Standard_Library/DCM/AEMS_FLOAT_TO_FXP_WITH_LIMIT: Internal implementation has Min/Max Limits. And the parameter "ByteSize" has been changed to "Output Fixed Point datatype".
  | 5. AEMS_Standard_Library/DCM/AEMS_FXP_TO_FLOAT: Data Type Conversion block is added in the implementation to take care of floating resolution.
  | 6. AEMS_Standard_Library/BIT_OPERATION/AEMS_CONVERT_TO_UNSIGNED_SI: New Block is added to convert signed integers to unsigned integers.
  | 7. AEMS_Standard_Library/BIT_OPERATION/AEMS_EXTRACT_BIT: New child library AEMS_CONVERT_TO_UNSIGNED_SI will be added if the Input data type is a signed integer.
  | 8. AEMS_Standard_Library/DCM/AEMS_TO_FXP_WITH_LIMIT: The parameter ‘Byte Size’ is replaced with ‘Output Fixed Point Datatype’ and a Data Type Conversion block is added at the input side.
  | 9. AEMS_Standard_Library/DEM/AEMS_DEM_REP_IUMPR_DEN_RELEASE & AEMS_Standard_Library/DEM/AEMS_DEM_REP_IUMPR_FAULTDETECT: AEMS_DEM_IUMPR block is split as two blocks.
  |    The following child library blocks in "AEMS_Standard_Library/SUB"
  |    AEMS_DEM_REP_IUMPR_DEN_RELEASE_1D
  |    AEMS_DEM_REP_IUMPR_DEN_RELEASE_2D
  |    AEMS_DEM_REP_IUMPR_DEN_RELEASE_8D
  |    AEMS_DEM_REP_IUMPR_FAULTDETECT_1D
  |    AEMS_DEM_REP_IUMPR_FAULTDETECT_2D
  |    AEMS_DEM_REP_IUMPR_FAULTDETECT_8D
  | 10. AEMS_Standard_Library/DCM/AEMS_DCM_DID_READDATA: Updated the block to read signed FXP. Parameter changed from Byte Size to DataType.
  | 11. AEMS_Standard_Library/DCM/AEMS_DCM_DID_WRITEDATA: Updated the block to support negative values & Existing bugs were removed. Parameter changed from Byte Size to DataType.
  | 12. AEMS_Standard_Library/SUB/AEMS_CONVERT_BUFFER_TO_FLP: Updated the block to support negative integer values. Parameter “Byte Size” changed to “DIDType”.
  | 13. AEMS_Standard_Library/SUB/AEMS_CONVERT_BYTE_TO_FLP: A new block created to convert byte data to float data, based on the resolution and offset.
  | 14. New blocks: (By Etienne)
  |        AEMS_Standard_Library/SUB/AEMS_DEM_SET_DTR_9DU
  |        AEMS_Standard_Library/SUB/AEMS_DEM_SET_EVENT_DSBL_9D
  |        AEMS_Standard_Library/SUB/AEMS_DEM_GET_EVENT_STS_9D
  |        AEMS_Standard_Library/SUB/AEMS_DEM_SET_EVENT_STS_9D
  |        AEMS_Standard_Library/SUB/AEMS_DEM_SET_EVENT_AVL_9D
  | 
  | 15. Modified blocks: (By Etienne)
  |        AEMS_Standard_Library/DEM/AEMS_DEM_READ_DATA_PID01
  |        AEMS_Standard_Library/DEM/AEMS_DEM_SET_DTR
  |        AEMS_Standard_Library/DEM/AEMS_DEM_SET_EVENT_DSBL
  |        AEMS_Standard_Library/DEM/AEMS_DEM_GET_EVENT_STS
  |        AEMS_Standard_Library/DEM/AEMS_DEM_SET_EVENT_STS
  |        AEMS_Standard_Library/DEM/AEMS_DEM_SET_EVENT_AVL
  |        AEMS_Standard_Library/SUB/AEMS_DEM_SET_EVENT_AVL_1D
  |        AEMS_Standard_Library/SUB/AEMS_DEM_SET_EVENT_AVL_2D
  |        AEMS_Standard_Library/SUB/AEMS_DEM_SET_EVENT_AVL_8D
  | 
  | 
  | 
  | AEMS_Standard_Library_02_10: by Thilagavathi, 11-12-2018
  | 1. Reversed the order of byte for the block "AEMS_DCM_DID_WRITEDATA" in the path "AEMS_Standard_Library/DCM/AEMS_DCM_DID_WRITEDATA"
  | 2. A new block added in the path "AEMS_Standard_Library/SPECIFIC/AEMS_SlopeSwitchExtern"
  | 3. Updated the constnat block parameter for the block "AEMS_INTERP" in the path "AEMS_Standard_Library/LOOKUP_TABLES/AEMS_INTERP"
  | 4. Added the Mask parameter(function mode) for the blocks "AEMS_FIM_GETFUNCTIONINHIBITION, AEMS_FIM_GET_FUNC_PMT_1D, AEMS_FIM_GET_FUNC_PMT_2D & AEMS_FIM_GETFUNCTIONPERMISSION"
  |     in the following path "AEMS_Standard_Library/DEM/AEMS_FIM_GETFUNCTIONINHIBITION" & "AEMS_Standard_Library/SUB/"
  | 5. Upadted data type for 18 Supplier call blocks in the path "AEMS_Standard_Library/SPECIFIC"
  | 6. Attribute string formate changed for the block "AEMS_DEM_COUNTER_BASED_DEBOUNCE" in path "AEMS_Standard_Library/DEM/AEMS_DEM_COUNTER_BASED_DEBOUNCE"
  | 7. Attribute string formate changed for the block "AEMS_DEM_TIME_BASED_DEBOUNCE" in path "AEMS_Standard_Library/DEM/AEMS_DEM_TIME_BASED_DEBOUNCE"
  | 8. changed the subsystem "DEM_SET_EVENT_AVL_E as atomic unit" for block "AEMS_DEM_SET_EVENT_AVL_1D" in the path "AEMS_Standard_Library/SUB/AEMS_DEM_SET_EVENT_AVL_1D"
  | 9. changed the subsystem "DEM_SET_EVENT_AVL_E as atomic unit" for block "AEMS_DEM_SET_EVENT_AVL_2D" in the path "AEMS_Standard_Library/SUB/AEMS_DEM_SET_EVENT_AVL_2D"
  | 10. changed the subsystem "DEM_SET_EVENT_AVL_E as atomic unit" for block "AEMS_DEM_SET_EVENT_AVL_8D" in the path "AEMS_Standard_Library/SUB/AEMS_DEM_SET_EVENT_AVL_8D"
  | 11. A new block "AEMS_FRAME_SUPERVISION" added in the path "AEMS_Standard_Library/COM/AEMS_FRAME_SUPERVISION"
  | 12. updated the block “AEMS_TIMER_H” to avoid the issue(“when timer is start incrementing / decrementing it is not taking the updated target counter value”) in AEMS_DEM_TIME_BASED_DEBOUNCE_THRSHOLD_DYN
  |      in the path "AEMS_Standard_Library/TIMER/AEMS_TIMER_H"
  | 13. Updated blocks "AEMS_DEM_TIME_BASED_DEBOUNCE_THRSHOLD_DYN & AEMS_DEM_COUNTER_BASED_DEBOUNCE_THRSHOLD_DYN" are added in the path "AEMS_Standard_Library/DEM"
  | 14. The following new blocks are added in the path "AEMS_Standard_Library/SUB"
  |       AEMS_DEM_TIME_BASED_DEBOUNCE_THRSHOLD_DYN_1D
  |       AEMS_DEM_TIME_BASED_DEBOUNCE_THRSHOLD_DYN_2D
  |       AEMS_DEM_TIME_BASED_DEBOUNCE_THRSHOLD_DYN_3D
  |       AEMS_DEM_TIME_BASED_DEBOUNCE_THRSHOLD_DYN_4D
  |       AEMS_DEM_TIME_BASED_DEBOUNCE_THRSHOLD_DYN_6D
  |       AEMS_DEM_TIME_BASED_DEBOUNCE_THRSHOLD_DYN_8D
  |       AEMS_DEM_COUNTER_BASED_DEBOUNCE_THRSHOLD_DYN_1D
  |       AEMS_DEM_COUNTER_BASED_DEBOUNCE_THRSHOLD_DYN_2D
  |       AEMS_DEM_COUNTER_BASED_DEBOUNCE_THRSHOLD_DYN_3D
  |       AEMS_DEM_COUNTER_BASED_DEBOUNCE_THRSHOLD_DYN_4D
  |       AEMS_DEM_COUNTER_BASED_DEBOUNCE_THRSHOLD_DYN_6D
  |       AEMS_DEM_COUNTER_BASED_DEBOUNCE_THRSHOLD_DYN_8D
  | 15. Updated the block "AEMS_DCM_DID_WRITEDATA" (replaced the block AEMS_NVM_WRITEONFLY by AEMS_NVM_WRITEONFLY_ENABLE) in the path "AEMS_Standard_Library/DCM/AEMS_DCM_DID_WRITEDATA"
  | 16. A new block "AEMS_NVM_WRITEONFLY_ENABLE" added in the path "AEMS_Standard_Library/MEM/AEMS_NVM_WRITEONFLY_ENABLE"
  | 17. A new block added in the path "AEMS_Standard_Library/COM/AEMS_REQUEST_COUNTER_SWITCH" (migrated from REMS)
  | 18. A new block added in the path "AEMS_Standard_Library/COM/AEMS_REQUEST_COUNTER" (migrated from REMS)
  | 
  | 
  | AEMS_Standard_Library_02_09: by Thilagavathi, 30-08-2018
  | 1. 84 Supplier call blocks are Migrated from REMS (SUPP_CALL_TQ_LIM, SUPPLIER_CALL_FFW & SUPPLIER_CALL_TIM category) and added in the path "AEMS_Standard_Library/SPECIFIC/"
  | 2. Reversed the order of byte for the block "AEMS_DCM_DID_READDATA" in the path "AEMS_Standard_Library/DCM/AEMS_DCM_DID_READDATA"
  | 3. The sample time is changed as '-1' for the block "AEMS_DEM_SET_EVENT_AVL" in the path "AEMS_Standard_Library/DEM/AEMS_DEM_SET_EVENT_AVL"
  | 4. A new block added in the path "AEMS_Standard_Library/DCM/AEMS_DCM_GETSESCTRLTYPE"
  | 5. A new block added in the path "AEMS_Standard_Library/MATH/AEMS_SQRT"
  | 
  | AEMS_Standard_Library_02_08: by Prabhakaran, 30-07-2018
  | 1. Update parameter Duration of Timer in miliseconde for block  in the path "AEMS_Standard_Library/DCM/AEMS_APP_REQUEST_IOCONTROL"
  | 2. Update parameter Duration of Timer (in seconde) for block  in the path "AEMS_Standard_Library/DCM/AEMS_APP_REQUEST_ROUTINE"
  | 3. The following supplier call block are added in the path "AEMS_Standard_Library/SPECIFIC/".
  |  - AEMS_SUPPLIER_CALL_ESTI_TIME_INJ
  |  - AEMS_SUPPLIER_CALL_FUEL_INJ_MIN
  |  - AEMS_SUPPLIER_CALL_PHI_MIN_ING
  |  - AEMS_SUPPLIER_CALL_SEPERATION_MIN_TIME
  |  - AEMS_SUPPLIER_CALL_TI_MIN_OK
  | 4. The following library blocks moved from DISCONTINUITIES to SPECIFIC Category as requiested by Naveen & NML
  |  - AEMS_AT_EHR - "AEMS_Standard_Library/DISCONTINUITIES/AEMS_AT_EHR"
  |  - AEMS_MULTIPORT_TIMESWITCH_CONFIG - "AEMS_Standard_Library/DISCONTINUITIES/AEMS_MULTIPORT_TIMESWITCH_CONFIG"
  |  - AEMS_AT_TUBE - "AEMS_Standard_Library/DISCONTINUITIES/AEMS_AT_TUBE"
  | 
  | AEMS_Standard_Library_02_07: by Thilagavathi, 17-07-2018
  | - A new block added in the path "AEMS_Standard_Library/DISCONTINUITIES/AEMS_AS_PADE"
  | - The block parameter 'DisableCoverage' is set to OFF in the following blocks to enable the coloring option while taking coverage.
  |   1. AEMS_Standard_Library/DISCRETE/AEMS_UNITDELAY_RESET_EXTERNALIC/FixPt_Logical_Operator,
  |   2. AEMS_Standard_Library/DISCRETE/AEMS_UNITDELAY_RESET_EXTERNALIC/FixPt_Logical_Operator1.
  | -A new block added in the path "AEMS_Standard_Library/DISCONTINUITIES/AEMS_AT_EHR"
  | -A new block added in the path "AEMS_Standard_Library/DISCONTINUITIES/AEMS_MULTIPORT_TIMESWITCH_CONFIG"
  | -A new block added in the path "AEMS_Standard_Library/DISCONTINUITIES/AEMS_AT_TUBE"
  | 
  | AEMS_Standard_Library_02_06: by Van-Cuong NGUYEN, 17-05-2018
  | 
  | AEMS_Standard_Library_02_05: by Van-Cuong NGUYEN, 27-03-2018
  | AEMS_Standard_Library/FILTER/AEMS_TAU_TO_FILTER_PARAM: Add block convert time constant to filter parameter, this is only used for filter block
  | AEMS_Standard_Library/DCM/AEMS_API_SUPPLIER_CALL: Add block API Supplier Call to use as interface with Supplier layer. It is not a functionnal block.
  | AEMS_Standard_Library/DCM/AEMS_TO_FXP_WITH_LIMIT: Change option convert from <<round>> to <<floor>> to respect MBDR.
  | AEMS_Standard_Library/DEM/AEMS_DEM_COUNTER_BASED_DEBOUNCE: Update parameter EventId such that block simulate without defining this parameter in workspace.
  | AEMS_Standard_Library/DEM/AEMS_DEM_COUNTER_BASED_DEBOUNCE_THRSHOLD_DYN: Update parameter EventId such that block simulate without defining this parameter in workspace.
  | AEMS_Standard_Library/DEM/AEMS_DEM_TIME_BASED_DEBOUNCE: Update parameter EventId such that block simulate without defining this parameter in workspace.
  | AEMS_Standard_Library/DEM/AEMS_DEM_TIME_BASED_DEBOUNCE_THRSHOLD_DYN: Update parameter EventId such that block simulate without defining this parameter in workspace.
  | AEMS_Standard_Library/DEM/AEMS_DEM_SET_EVENT_AVL: Update parameter EventId such that block simulate without defining this parameter in workspace.
  | 
  | AEMS_Standard_Library_02_04: by Van-Cuong NGUYEN, 14-03-2018
  | AEMS_DEM_TIME_BASED_DEBOUNCE_THRSHOLD_DYN: add in DEM category new block for time based debounce with threshold dynamic and for Nissan uses only
  | AEMS_DEM_COUNTER_BASED_DEBOUNCE_THRSHOLD_DYN: add in DEM category new block for counter based debounce with threshold dynamic and for Nissan uses only
  | AEMS_DCM_DID_READDATA: correct problem of simulation for inport boolean and add inport name in mask for each inport
  | AEMS_DCM_DID_WRITEDATA: correct problem of simulation for inport boolean and add inport name in mask for each inport
  | 
  | AEMS_Standard_Library_02_03: by Van-Cuong NGUYEN, 06-02-2018
  | DEM Blocks
  | AEMS_Standard_Library/DEM/AEMS_DEM_GET_INDICATOR_STS
  | AEMS_Standard_Library/DEM/AEMS_DEM_READ_DATA_PID01
  | AEMS_Standard_Library/DEM/AEMS_DEM_REP_IUMPR
  | AEMS_Standard_Library/DEM/AEMS_DEM_SET_DTR
  | AEMS_Standard_Library/DEM/AEMS_DEM_SET_ENBL_COND
  | AEMS_Standard_Library/DEM/AEMS_DEM_SET_EVENT_DSBL
  | AEMS_Standard_Library/DEM/AEMS_DEM_SET_EVENT_STS
  | AEMS_Standard_Library/DEM/AEMS_DEM_SET_IUMPR_DCOND
  | AEMS_Standard_Library/DEM/AEMS_DEM_SET_OPCYC_STE
  | AEMS_Standard_Library/DEM/AEMS_DEM_SET_PFC_CYC_QUALD
  | AEMS_Standard_Library/DEM/AEMS_DEM_SET_EVENT_AVL
  | AEMS_Standard_Library/DEM/AEMS_DEM_GET_EVENT_STS
  | DCM Blocks
  | AEMS_Standard_Library/DCM/AEMS_APP_DID_WRITEDATA
  | AEMS_Standard_Library/DCM/AEMS_APP_REQUEST_IOCONTROL
  | AEMS_Standard_Library/DCM/AEMS_APP_REQUEST_ROUTINE
  | AEMS_Standard_Library/DCM/AEMS_DCM_DID_READDATA
  | AEMS_Standard_Library/DCM/AEMS_DCM_DID_WRITEDATA
  | AEMS_Standard_Library/DCM/AEMS_DCM_IO_RETURN_CONTROL_TO_ECU
  | AEMS_Standard_Library/DCM/AEMS_DCM_IO_SHORT_TERM_ADJUSTEMENT
  | AEMS_Standard_Library/DCM/AEMS_DCM_REQUEST_RESULT
  | AEMS_Standard_Library/DCM/AEMS_DCM_START_ROUTINE
  | AEMS_Standard_Library/DCM/AEMS_DCM_STOP_ROUTINE
  | 
  | AEMS_Standard_Library_02_02: by Van-Cuong NGUYEN, 24-01-2018
  | DEM: Remove block:
  | AEMS_INVOKE_AUTOSAR_SERVER_OPERATION
  | DISCONTINUOUS: Add blocks
  | AEMS_SLOPE_SWITCH_3INPUTS
  | AEMS_SLOPE_SWITCH_6INPUTS
  | 
  | AEMS_Standard_Library_02_01: by Van-Cuong NGUYEN, 16-01-2018
  | MEM: AEMS_NVM_WRITEONFLY
  | DEM: List of blocks added
  | AEMS_DEM_SET_EVENT_AVL
  | AEMS_DEM_GET_EVENT_STS
  | AEMS_DEM_COUNTER_BASED_DEBOUNCE
  | AEMS_DEM_TIME_BASED_DEBOUNCE
  | FIM: AEMS_FIM_GETFUNCTIONINHIBITION
  | DISCONTINUOUS: Change setting StateWhenEnable from Reset to Held to have a coherence with Renault blocks and functionality
  | AEMS_SLOPE_SWITCH
  | AEMS_SLOPE_SWITCH_4INPUTS
  | AEMS_SLOPE_SWITCH_8INPUTS
  | 
  | AEMS_Standard_Library_02_00: by Van-Cuong NGUYEN, 27-11-2017
  | Convergence of Renault/Nissan blocks to AEMS blocks based on AUTOSAR standard.
  | Three groups of blocks: Standard blocks which have commun functionality defined by AUTOSAR standard,
  | specific Nissan block  and specific Renault blocks.
  | 
  | AEMS_Standard_Library_01_00:by Van-Cuong NGUYEN, 10-02-2017
  | Initial version: Convergence of Renault/Nissan blocks to AEMS blocks.
settings DataIOCC: LimitDataPoints=on  SaveFormat=Array  SignalLoggingSaveFormat=ModelDataLogs
settings OptimizationCC: BlockReduction=off  BooleanDataType=off  LifeSpan=inf
settings DebuggingCC: SaveWithParameterizedLinksMsg=none  UnderspecifiedInitializationDetection=Classic  MergeDetectMultiDrivingBlocksExec=none  SignalResolutionControl=TryResolveAllWithWarning  MultiTaskDSMMsg=warning  MultiTaskCondExecSysMsg=none  StrictBusMsg=None  SFUnexpectedBacktrackingDiag=warning  SFNoUnconditionalDefaultTransitionDiag=warning  SFExecutionAtInitializationDiag=none
settings HardwareCC: ProdBitPerPointer=32  ProdBitPerSizeT=32  ProdBitPerPtrDiffT=32  ProdLargestAtomicFloat=None  ProdIntDivRoundTo=Undefined  ProdEndianess=Unspecified  ProdWordSize=32  ProdHWDeviceType=32-bit Generic  TargetUnknown=on
settings ModelReferenceCC: PropagateSignalLabelsOutOfModel=off
settings GRTTargetCC: TargetLangStandard=C89/C90 (ANSI)  GeneratePreprocessorConditionals=Disable all
settings ConfigComp: CovMetricSettings=dw  CovHtmlReporting=on  CovSaveCumulativeToWorkspaceVar=on  CovSaveSingleToWorkspaceVar=on  CovExternalEMLEnable=off

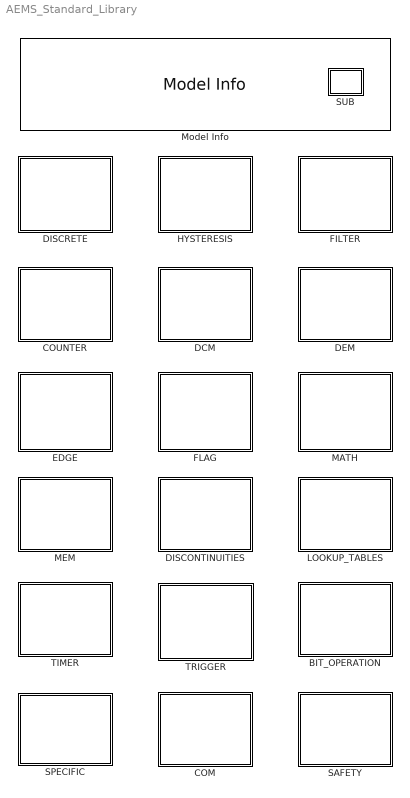
== system AEMS_Standard_Library ==
  BIT_OPERATION : Subsystem
  COM : Subsystem
  COUNTER : Subsystem
  DCM : Subsystem
  DEM : Subsystem
  DISCONTINUITIES : Subsystem
  DISCRETE : Subsystem
  EDGE : Subsystem
  FILTER : Subsystem
  FLAG : Subsystem
  HYSTERESIS : Subsystem
  LOOKUP_TABLES : Subsystem
  MATH : Subsystem
  MEM : Subsystem
  Model Info : simulink/Model-Wide Utilities/Model Info  Frame=on  DisplayStringWithTags=|  HorizontalTextAlignment=Center  LeftAlignmentValue=0.5  SourceBlockDiagram=AEMS_Standard_Library  TagMaxNumber=20
      | Model Info
      | %<ModelVersion>
      | Editor: %<LastModifiedBy>
      | Last modified: %<LastModificationDate>
  SAFETY : Subsystem
  SPECIFIC : Subsystem
  SUB : Subsystem
  TIMER : Subsystem
  TRIGGER : Subsystem
